simulink model "Model4"  (R2022b)
settings: Solver=FixedStepDiscrete  StartTime=0.0  StopTime=60  FixedStep=T  RelTol=1e-3
undefined symbols (not defined in the file or in its folder): K_d
libraries: cstblocks x2
settings Model: Creator=Sahil Gaurkar  LastModifiedBy=Sahil Gaurkar

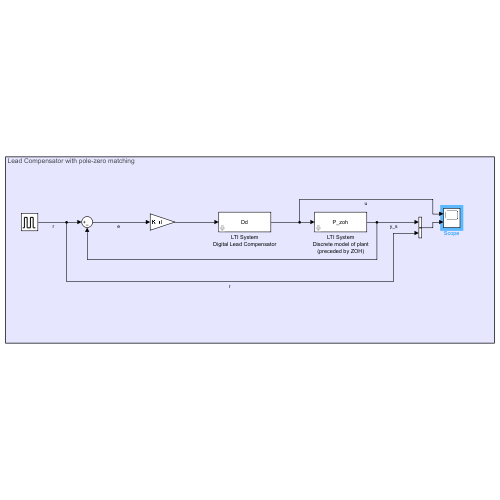
[thumbnail: Simulink's stored preview of the top-level diagram]
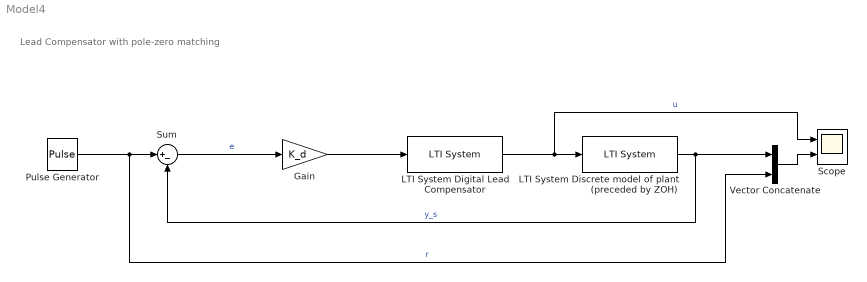
== system Model4 ==
  note: Lead Compensator with pole-zero matching
  Gain : Gain  Gain=K_d
  LTI System Digital Lead Compensator : cstblocks/LTI System  sys=Dd  IC=[]
  LTI System Discrete model of plant (preceded by ZOH) : cstblocks/LTI System  sys=P_zoh  IC=[]
  Pulse Generator : DiscretePulseGenerator  PulseType=Time based  Period=10  PulseWidth=50
  Scope : Scope  NumInputPorts=2
  Sum : Sum  Inputs=|+-
  Vector Concatenate : Concatenate
  wires:
  Vector Concatenate/1 -> Scope/2
  LTI System Digital Lead Compensator/1 -> Scope/1, LTI System Discrete model of plant (preceded by ZOH)/1  "u"
  Pulse Generator/1 -> Vector Concatenate/2, Sum/1  "r"
  Sum/1 -> Gain/1  "e"
  Gain/1 -> LTI System Digital Lead Compensator/1
  LTI System Discrete model of plant (preceded by ZOH)/1 -> Vector Concatenate/1, Sum/2  "y_s"
